simulink model "simulink6"  (R2017a)
settings: Solver=VariableStepAuto  StartTime=0.0  StopTime=10.0  RelTol=1e-3
libraries: cstblocks x5
settings Model: Creator=Night_Fury  LastModifiedBy=Havoc

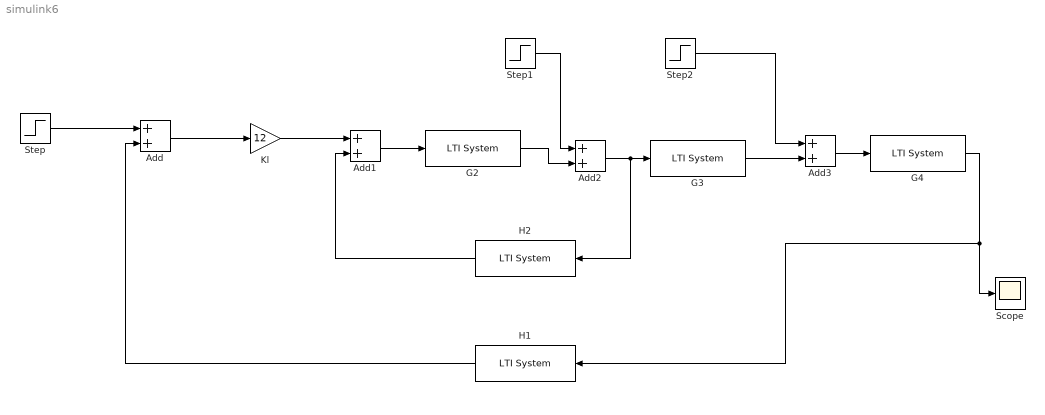
== system simulink6 ==
  Add{,1..3} (4 alike) : Sum
  G2 : cstblocks/LTI System  sys=tf([1],[1 1 8])  IC=[]
  G3 : cstblocks/LTI System  sys=tf([20],[1 1])  IC=[]
  G4 : cstblocks/LTI System  sys=tf([10],[2 1])  IC=[]
  H1 : cstblocks/LTI System  sys=tf([1],[1 1])  IC=[]
  H2 : cstblocks/LTI System  sys=tf(5,[1 0])  IC=[]
  "Kl " : Gain  Gain=12
  Scope : Scope
  Step : Step  SampleTime=0
  Step1 : Step  SampleTime=0
  Step2 : Step  SampleTime=0
  wires:
  Step/1 -> Add/1
  Add/1 -> "Kl "/1
  G3/1 -> Add3/2
  G4/1 -> H1/1, Scope/1
  "Kl "/1 -> Add1/1
  Add1/1 -> G2/1
  G2/1 -> Add2/2
  Add2/1 -> H2/1, G3/1
  Add3/1 -> G4/1
  Step1/1 -> Add2/1
  Step2/1 -> Add3/1
  H1/1 -> Add/2
  H2/1 -> Add1/2
